simulink model "lab08q1_b"  (Simulink 6.6)
settings: Solver=ode45  StartTime=0.0  StopTime=0.2  RelTol=1e-3
InitFcn:
  | R1 = 5*10^3 %% AQUI ENTRA O VALOR DE R1 DA TABELA DA QUESTAO 01 LETRA B...
  | 
  | R2 = 60*10^3;
  | R3 = 5*10^3;
  | R4 = 5*10^3;
  | k  = R3/R4;
  | 
  | C1 = 250*10^(-9);
  | C2 = C1;
  | 
  | A = [((-1/(R1*C1))-(1/(R2*C1))) ((1+k)*(1/(R1*C1))+k*(1/(R2*C1)));(-1/(R2*C2)) (1/(R2*C2))*k]
  | 
  | B = [-(1/(R1*C1));0]
  | 
  | C = [0 (1+k);1 0;0 1]
  | 
  | D = [0;0;0]
settings Model: Creator=ALUNO  LastModifiedBy=Rawlinson
settings GRTTargetCC: TargetFcnLib=ansi_tfl_table_tmw.mat

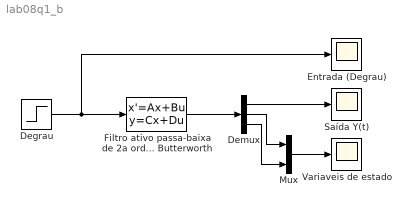
== system lab08q1_b ==
  Degrau : Step  Time=0  SampleTime=0
  Demux : Demux  Outputs=3
  Entrada (Degrau) : Scope
      settings: SaveName=ScopeData2
  Filtro ativo passa-baixa de 2a ordem Butterworth : StateSpace  A=A  B=B  C=C  D=D
  Mux : Mux  Inputs=2
  Saída Y(t) : Scope
      settings: TimeRange=0.2  YMin=0  YMax=2.5
  Variaveis de estado : Scope
  wires:
  Degrau/1 -> Filtro ativo passa-baixa de 2a ordem Butterworth/1, Entrada (Degrau)/1
  Filtro ativo passa-baixa de 2a ordem Butterworth/1 -> Demux/1
  Mux/1 -> Variaveis de estado/1
  Demux/1 -> Saída Y(t)/1
  Demux/2 -> Mux/1
  Demux/3 -> Mux/2
